simulink model "sim_sistema_3"  (Simulink 8.9)
settings: Solver=ode3  StartTime=0.0  StopTime=20  FixedStep=1e-4  RelTol=1e-3  EnableMultiTasking=on
values from neighbouring files (symbols this model uses):
  A = [-5 1 0;0 -2 1;0 0 -1]    [sistema_3.m]    (also in sistema_3_2.m)
  B = [0 0 1]'    [sistema_3.m]    (also in sistema_3_2.m)
  C = [1 0 0; 0 1 0; 0 0 1]    [sistema_3.m]    (also in sistema_3_2.m = [1 0 0])
  D = [0 0 0]'    [sistema_3.m]
  K = acker(Ac,Bc,J)    [sistema_3.m]    (also in sistema_3_2.m)
settings Model: Creator=taniel.franklin  LastModifiedBy=filip
settings OptimizationCC: ExpressionDepthLimit=2147483647
settings DebuggingCC: SolverPrmCheckMsg=warning

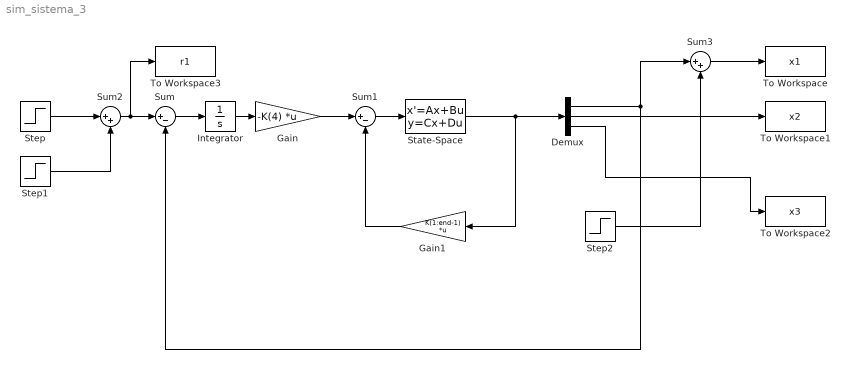
== system sim_sistema_3 ==
  Demux : Demux  Outputs=3
  Gain : Gain  Gain=-K(4)  Multiplication=Matrix(K*u)
  Gain1 : Gain  Gain=K(1:end-1)  Multiplication=Matrix(K*u)
  Integrator : Integrator
  State-Space : StateSpace  A=A  B=B  C=C  D=D  X0=[0 0 0]'
  Step : Step  Time=0.1  SampleTime=0
  Step1 : Step  Time=8  SampleTime=0
  Step2 : Step  Time=14  SampleTime=0
  Sum : Sum  Inputs=|+-
  Sum1 : Sum  Inputs=|+-
  Sum2 : Sum  Inputs=|++
  Sum3 : Sum  Inputs=|++
  To Workspace : ToWorkspace  VariableName=x1  SaveFormat=Structure With Time  SampleTime=-1
  To Workspace1 : ToWorkspace  VariableName=x2  SaveFormat=Structure With Time  SampleTime=-1
  To Workspace2 : ToWorkspace  VariableName=x3  SaveFormat=Structure With Time  SampleTime=-1
  To Workspace3 : ToWorkspace  VariableName=r1  SaveFormat=Structure With Time  SampleTime=-1
  wires:
  State-Space/1 -> Demux/1, Gain1/1
  Demux/2 -> To Workspace1/1
  Sum/1 -> Integrator/1
  Sum1/1 -> State-Space/1
  Step/1 -> Sum2/1
  Step1/1 -> Sum2/2
  Sum2/1 -> Sum/1, To Workspace3/1
  Demux/1 -> Sum3/1, Sum/2
  Gain1/1 -> Sum1/2
  Integrator/1 -> Gain/1
  Gain/1 -> Sum1/1
  Demux/3 -> To Workspace2/1
  Sum3/1 -> To Workspace/1
  Step2/1 -> Sum3/2
